simulink library "Autonomous_lib"  (R2023b)
settings: Solver=VariableStepAuto  StartTime=0.0  StopTime=10.0  RelTol=1e-3
settings Model: Creator=FIRSTMentor  LastModifiedBy=ander

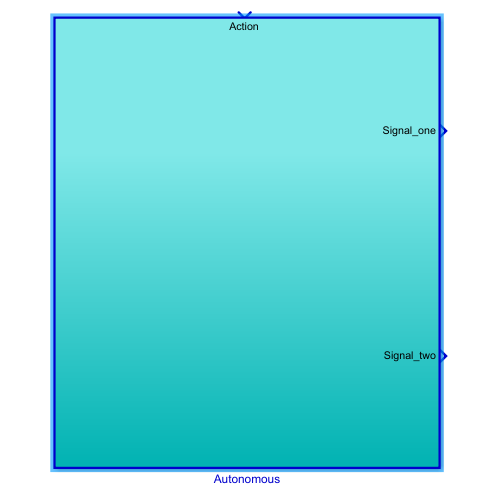
[thumbnail: Simulink's stored preview of the top-level diagram]
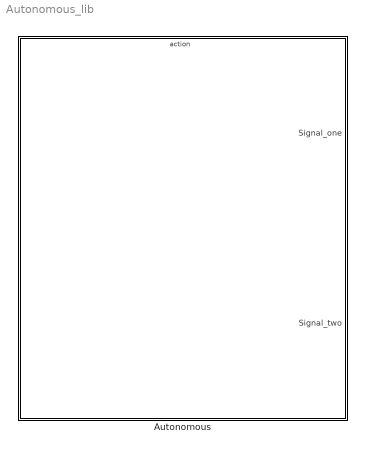
== system Autonomous_lib ==
  Autonomous : Subsystem  TreatAsAtomicUnit=on

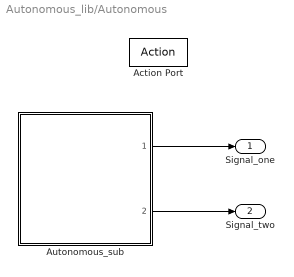
== system Autonomous_lib/Autonomous ==
  Action Port : ActionPort  InitializeStates=reset
  Autonomous_sub : Subsystem  ReferencedSubsystem=Autonomous_sub
  Signal_one : Outport
  Signal_two : Outport  Port=2
  wires:
  Autonomous_sub/1 -> Signal_one/1
  Autonomous_sub/2 -> Signal_two/1
